simulink model "vslipsl_sim"  (R2022b)
settings: Solver=ode45  StartTime=0.0  StopTime=Tf  FixedStep=1e-3  RelTol=1e-11  AbsTol=1e-11
values from neighbouring files (symbols this model uses):
  flag_dist = 0    [main.m]    (also in main_slip_w_sw_leg.m)
  gains = [gain.K_p; gain.K_d; gain.K_p_sw; gain.K_d_sw; gain.K_p_ds; gain.K_d_ds; gain.K_v_ds]    [main.m]    (also in main_slip_w_sw_leg.m)
  init_cond = [x_M_init; y_M_init; theta_init; r_init; x_CoM_init; y_CoM_init; dx_M_init; dy_M_init; dtheta_init; dr_init; dx_CoM_init; dy_CoM_init]    [main.m]    (also in main_slip_w_sw_leg.m)
  init_f_record = 0    [main.m]    (also in main_slip_w_sw_leg.m)
  init_flag = [1; dc.col_param.foot; -dc.col_param.footPlus; x_M_init; x_CoM_ss_init; flag_ref_ob]    [main.m]    (also in main_slip_w_sw_leg.m = [1; dc.col_param.foot; -dc.col_param.footPlus; x_M_init; x_C)
  param = [L0_ss; k0_ss; m_M; m_swLeg; m_swFoot; I_swLeg; I_swFoot; L_thigh; k_swFoot; k_swLeg; theta_s0; r_s0; g; L0_ds; k0_ds]    [main.m]    (also in main_slip_w_sw_leg.m)
  ref_star_ds = [ref_star.ds.x_CoM_star,      ref_star.ds.y_CoM_star, ref_star.ds.dx_CoM_star,      ref_star.ds.del_y_CoM_star, ref_star.ds.del_dx_CoM_star,      ref_star.ds.del2_y_CoM_star]    [main.m]    (also in main_slip_w_sw_leg.m)
  ref_star_ss = [ref_star.ss.x_M_star,      ref_star.ss.y_M_star, ref_star.ss.x_swFoot_star, ref_star.ss.y_swFoot_star,      ref_star.ss.del_y_M_star, ref_star.ss.del_x_swFoot_star, ref_star.ss.del_y_swFoot_star,      ref_star.ss.del2_y_M_star, ref_star.ss.del2_x_swFoot_star, ref_star.ss.del2_y_swFoot_star,      ref_star.ss.x_CoM_star]    [main.m]    (also in main_slip_w_sw_leg.m)
  sample_time = 0.001    [main.m]    (also in main_slip_w_sw_leg.m)
libraries: simulink x1
settings Model: SimulationMode=accelerator  Creator=Pelit  LastModifiedBy=mmpel
settings SolverCC: InitialStep=1e-5  AlgebraicLoopSolver=TrustRegion
settings DataIOCC: ReturnWorkspaceOutputs=off
settings DebuggingCC: UnconnectedInputMsg=warning  UnconnectedOutputMsg=warning  UnconnectedLineMsg=warning  SFMachineParentedDataDiag=warning  ArithmeticOperatorsInVariantConditions=warning
settings ModelReferenceCC: EnableRefExpFcnMdlSchedulingChecks=on
settings SFSimCC: SimUseLocalCustomCode=off  CustomCodeUndefinedFunction=UseInterfaceOnly
settings RTWCC: RTWUseLocalCustomCode=off  DLArmComputeVersion=19.05

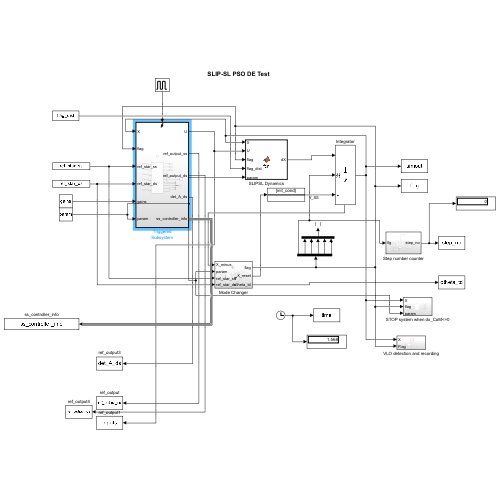
[thumbnail: Simulink's stored preview of the top-level diagram]
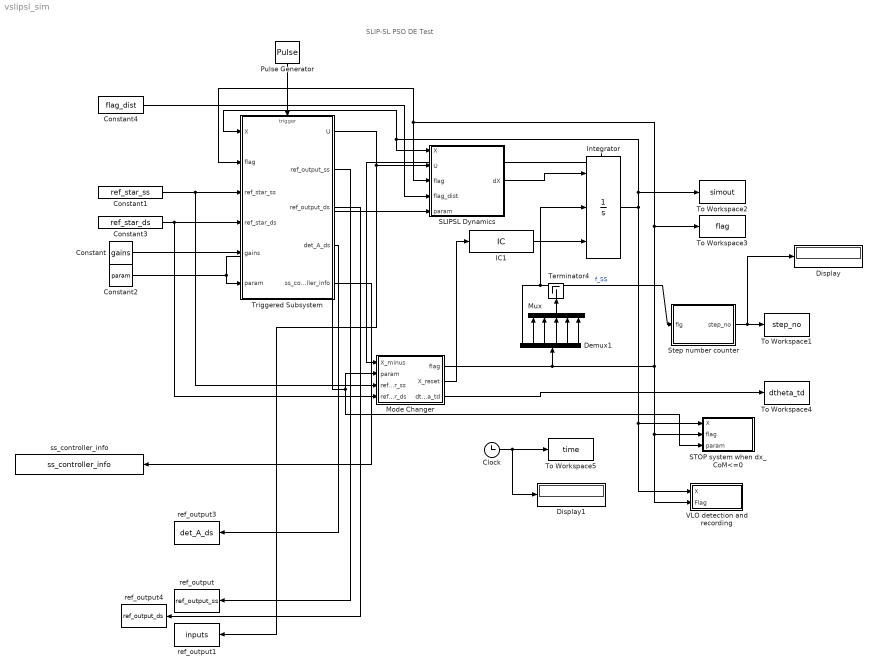
== system vslipsl_sim ==
  note: SLIP-SL PSO DE Test
  Clock : Clock
  Constant : Constant  Value=gains
  Constant1 : Constant  Value=ref_star_ss
  Constant2 : Constant  Value=param
  Constant3 : Constant  Value=ref_star_ds
  Constant4 : Constant  Value=flag_dist
  Demux1 : Demux  Outputs=6
  Display : Display
  Display1 : Display
  IC1 : InitialCondition  Value=init_cond
  Integrator : Integrator  ExternalReset=either  InitialConditionSource=external  ShowStatePort=on
  Mode Changer : Subsystem
  Mux : Mux  Inputs=5
  Pulse Generator : DiscretePulseGenerator  PulseType=Time based  Period=1e-3  PulseWidth=5
  SLIPSL Dynamics : MATLAB Function  TreatAsAtomicUnit=on
  STOP system when dx_CoM<=0 : Subsystem
  Step number counter : Subsystem
  Terminator4 : Terminator
  To Workspace1 : ToWorkspace  VariableName=step_no  SampleTime=sample_time
  To Workspace2 : ToWorkspace  VariableName=simout  SampleTime=sample_time
  To Workspace3 : ToWorkspace  VariableName=flag  SampleTime=sample_time
  To Workspace4 : ToWorkspace  VariableName=dtheta_td  SampleTime=sample_time
  To Workspace5 : ToWorkspace  VariableName=time  SampleTime=sample_time
  Triggered Subsystem : Subsystem  TreatAsAtomicUnit=on
  VLO detection and recording : Subsystem
  ref_output : ToWorkspace  VariableName=ref_output_ss  SampleTime=sample_time
  ref_output1 : ToWorkspace  VariableName=inputs  SampleTime=sample_time
  ref_output3 : ToWorkspace  VariableName=det_A_ds  SampleTime=sample_time
  ref_output4 : ToWorkspace  VariableName=ref_output_ds  SampleTime=sample_time
  ss_controller_info : ToWorkspace  VariableName=ss_controller_info  SaveFormat=Timeseries  SampleTime=sample_time
  wires:
  SLIPSL Dynamics/1(dX) -> Integrator/1
  Mode Changer/1(flag) -> Demux1/1, Triggered Subsystem/2(flag), SLIPSL Dynamics/3(flag), To Workspace3/1, VLO detection and recording/2(Flag), STOP system when dx_CoM<=0/2(flag)
  Constant2/1 -> SLIPSL Dynamics/5(param), STOP system when dx_CoM<=0/3(param), Mode Changer/2("param "), Triggered Subsystem/6(param)
  Mode Changer/2(X_reset) -> IC1/1
  Integrator/1 -> VLO detection and recording/1(X), STOP system when dx_CoM<=0/1(X), To Workspace2/1, Triggered Subsystem/1(X), SLIPSL Dynamics/1(X)
  IC1/1 -> Integrator/3
  Demux1/1 -> Step number counter/1(flg), Integrator/2  "f_SS"
  Integrator/State -> Mode Changer/1(X_minus)
  Step number counter/1(step_no) -> Display/1, To Workspace1/1
  Mode Changer/3(dtheta_td) -> To Workspace4/1
  Clock/1 -> Display1/1, To Workspace5/1
  Constant1/1 -> Mode Changer/3(ref_star_ss), Triggered Subsystem/3(ref_star_ss)
  Triggered Subsystem/1(U) -> ref_output1/1, SLIPSL Dynamics/2(U)
  Triggered Subsystem/2(ref_output_ss) -> ref_output/1
  Constant3/1 -> Mode Changer/4(ref_star_ds), Triggered Subsystem/4(ref_star_ds)
  Triggered Subsystem/3(ref_output_ds) -> ref_output4/1
  Constant/1 -> Triggered Subsystem/5(gains)
  Constant4/1 -> SLIPSL Dynamics/4(flag_dist)
  Pulse Generator/1 -> Triggered Subsystem/Trigger
  Triggered Subsystem/4(det_A_ds) -> ref_output3/1
  Demux1/2 -> Mux/1
  Demux1/3 -> Mux/2
  Demux1/4 -> Mux/3
  Demux1/5 -> Mux/4
  Demux1/6 -> Mux/5
  Mux/1 -> Terminator4/1
  Triggered Subsystem/5(ss_controller_info) -> ss_controller_info/1

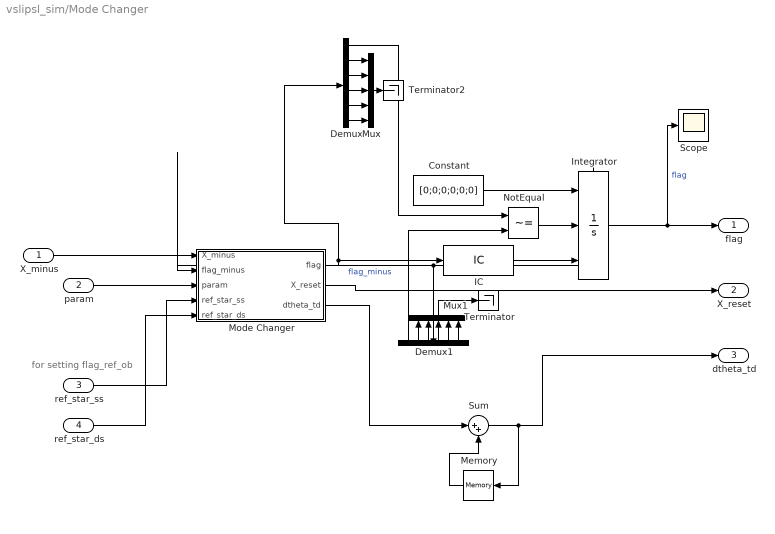
== system vslipsl_sim/Mode Changer ==
  note: for setting flag_ref_ob
  X_minus : Inport
  "param " : Inport  Port=2
  ref_star_ss : Inport  Port=3
  ref_star_ds : Inport  Port=4
  Constant : Constant  Value=[0;0;0;0;0;0]
  Demux : Demux  Outputs=6
  Demux1 : Demux  Outputs=6
  IC : InitialCondition  Value=init_flag
  Integrator : Integrator  ExternalReset=rising  InitialConditionSource=external  ShowStatePort=on
  Memory : Memory
  Mode Changer : MATLAB Function  TreatAsAtomicUnit=on
  Mux : Mux  Inputs=5
  Mux1 : Mux  Inputs=5
  NotEqual : RelationalOperator  Operator=~=  OutDataTypeStr=boolean  RndMeth=Simplest  InputSameDT=off
  Scope : Scope
  Sum : Sum  Inputs=|++
  Terminator : Terminator
  Terminator2 : Terminator
  flag : Outport  VectorParamsAs1DForOutWhenUnconnected=off
  X_reset : Outport  Port=2  VectorParamsAs1DForOutWhenUnconnected=off
  dtheta_td : Outport  Port=3  VectorParamsAs1DForOutWhenUnconnected=off
  wires:
  X_minus/1 -> Mode Changer/1(X_minus)
  IC/1 -> Integrator/3
  Integrator/State -> Mode Changer/2(flag_minus), Demux1/1  "flag_minus"
  "param "/1 -> Mode Changer/3(param)
  Mode Changer/1(flag) -> IC/1, Demux/1
  Constant/1 -> Integrator/1
  NotEqual/1 -> Integrator/2
  Integrator/1 -> Scope/1, flag/1  "flag"
  Mode Changer/2(X_reset) -> X_reset/1
  Mode Changer/3(dtheta_td) -> Sum/1
  Memory/1 -> Sum/2
  Sum/1 -> Memory/1, dtheta_td/1
  Demux1/1 -> NotEqual/2
  ref_star_ss/1 -> Mode Changer/4(ref_star_ss)
  ref_star_ds/1 -> Mode Changer/5(ref_star_ds)
  Demux/6 -> Mux/5
  Demux/5 -> Mux/4
  Demux/4 -> Mux/3
  Demux/3 -> Mux/2
  Demux/2 -> Mux/1
  Mux/1 -> Terminator2/1
  Demux/1 -> NotEqual/1
  Demux1/2 -> Mux1/1
  Demux1/3 -> Mux1/2
  Demux1/4 -> Mux1/3
  Demux1/5 -> Mux1/4
  Demux1/6 -> Mux1/5
  Mux1/1 -> Terminator/1

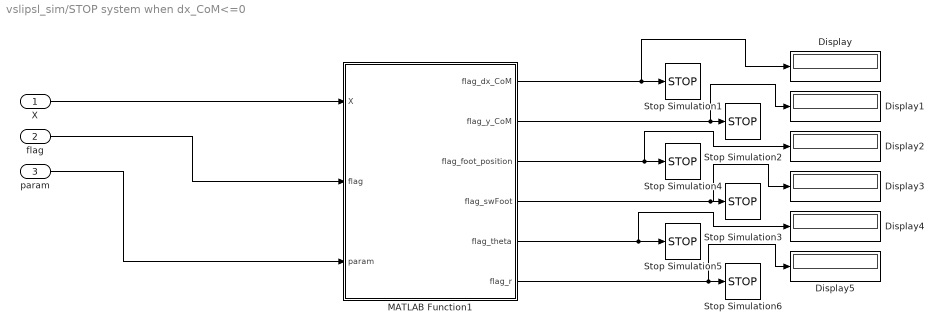
== system vslipsl_sim/STOP system when dx_CoM<=0 ==
  X : Inport
  flag : Inport  Port=2
  param : Inport  Port=3
  Display{,1..5} (6 alike) : Display
  MATLAB Function1 : MATLAB Function  TreatAsAtomicUnit=on
  Stop Simulation{1..6} (6 alike) : Stop
  wires:
  X/1 -> MATLAB Function1/1(X)
  MATLAB Function1/4(flag_swFoot) -> Display3/1, Stop Simulation3/1
  flag/1 -> MATLAB Function1/2(flag)
  param/1 -> MATLAB Function1/3(param)
  MATLAB Function1/1(flag_dx_CoM) -> Display/1, Stop Simulation1/1
  MATLAB Function1/2(flag_y_CoM) -> Display1/1, Stop Simulation2/1
  MATLAB Function1/3(flag_foot_position) -> Display2/1, Stop Simulation4/1
  MATLAB Function1/5(flag_theta) -> Display4/1, Stop Simulation5/1
  MATLAB Function1/6(flag_r) -> Display5/1, Stop Simulation6/1

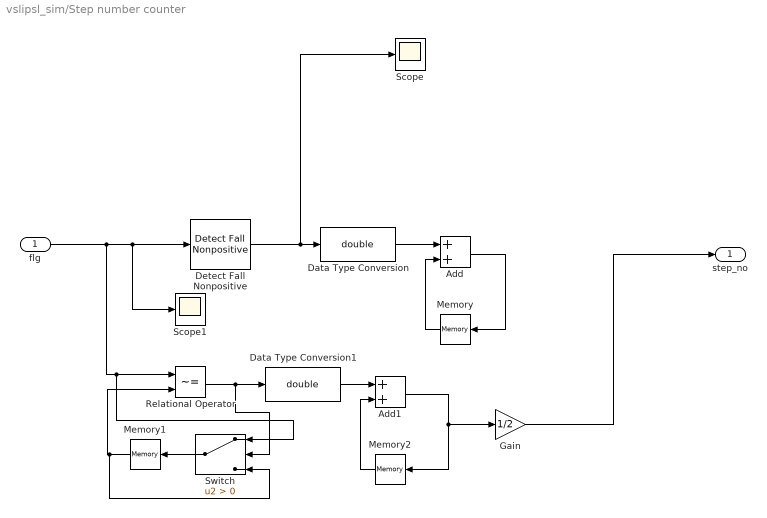
== system vslipsl_sim/Step number counter ==
  flg : Inport  SampleTime=sample_time
  Add : Sum
  Add1 : Sum
  Data Type Conversion : DataTypeConversion  OutDataTypeStr=double  SaturateOnIntegerOverflow=off  RndMeth=Floor
  Data Type Conversion1 : DataTypeConversion  OutDataTypeStr=double  SaturateOnIntegerOverflow=off  RndMeth=Floor
  Detect Fall Nonpositive : simulink/Logic and Bit Operations/Detect Fall Nonpositive  vinit=1  InputProcessing=Columns as channels (frame based)  OutDataTypeStr=boolean
  Gain : Gain  Gain=1/2
  Memory : Memory  InheritSampleTime=on
  Memory1 : Memory  InitialCondition=1  InheritSampleTime=on
  Memory2 : Memory  InheritSampleTime=on
  Relational Operator : RelationalOperator  Operator=~=  OutDataTypeStr=boolean  RndMeth=Simplest  InputSameDT=off
  Scope : Scope
  Scope1 : Scope
  Switch : Switch  Criteria=u2 > Threshold  SaturateOnIntegerOverflow=off  InputSameDT=off
  step_no : Outport  VectorParamsAs1DForOutWhenUnconnected=off
  wires:
  Add/1 -> Memory/1
  Memory/1 -> Add/2
  Detect Fall Nonpositive/1 -> Scope/1, Data Type Conversion/1
  Data Type Conversion/1 -> Add/1
  Memory1/1 -> Switch/3, Relational Operator/2
  Memory2/1 -> Add1/2
  Add1/1 -> Gain/1, Memory2/1
  Relational Operator/1 -> Switch/2, Data Type Conversion1/1
  Data Type Conversion1/1 -> Add1/1
  Switch/1 -> Memory1/1
  flg/1 -> Switch/1, Relational Operator/1, Detect Fall Nonpositive/1, Scope1/1
  Gain/1 -> step_no/1

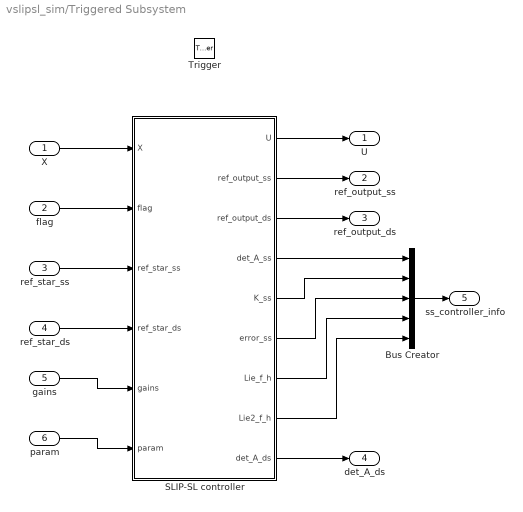
== system vslipsl_sim/Triggered Subsystem ==
  X : Inport
  flag : Inport  Port=2
  ref_star_ss : Inport  Port=3
  ref_star_ds : Inport  Port=4
  gains : Inport  Port=5
  param : Inport  Port=6
  Trigger : TriggerPort  VariantControl=Variant
  Bus Creator : BusCreator  Inputs=5
  SLIP-SL controller : MATLAB Function  TreatAsAtomicUnit=on
  U : Outport
  ref_output_ss : Outport  Port=2
  ref_output_ds : Outport  Port=3
  det_A_ds : Outport  Port=4
  ss_controller_info : Outport  Port=5
  wires:
  X/1 -> SLIP-SL controller/1(X)
  flag/1 -> SLIP-SL controller/2(flag)
  ref_star_ss/1 -> SLIP-SL controller/3(ref_star_ss)
  ref_star_ds/1 -> SLIP-SL controller/4(ref_star_ds)
  gains/1 -> SLIP-SL controller/5(gains)
  param/1 -> SLIP-SL controller/6(param)
  SLIP-SL controller/1(U) -> U/1
  SLIP-SL controller/2(ref_output_ss) -> ref_output_ss/1
  SLIP-SL controller/3(ref_output_ds) -> ref_output_ds/1
  SLIP-SL controller/4(det_A_ss) -> Bus Creator/1
  SLIP-SL controller/9(det_A_ds) -> det_A_ds/1
  Bus Creator/1 -> ss_controller_info/1
  SLIP-SL controller/5(K_ss) -> Bus Creator/2
  SLIP-SL controller/6(error_ss) -> Bus Creator/3
  SLIP-SL controller/7(Lie_f_h) -> Bus Creator/4
  SLIP-SL controller/8(Lie2_f_h) -> Bus Creator/5

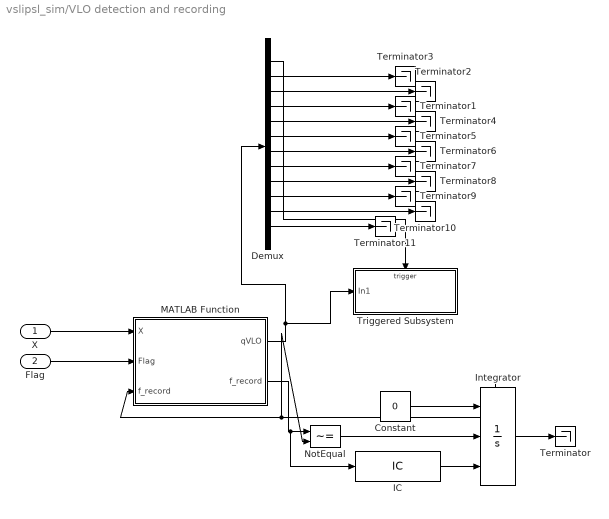
== system vslipsl_sim/VLO detection and recording ==
  X : Inport
  Flag : Inport  Port=2
  Constant : Constant  Value=0
  Demux : Demux  Outputs=12
  IC : InitialCondition  Value=init_f_record
  Integrator : Integrator  ExternalReset=rising  InitialConditionSource=external  ShowStatePort=on
  MATLAB Function : MATLAB Function  TreatAsAtomicUnit=on
  NotEqual : RelationalOperator  Operator=~=  OutDataTypeStr=boolean  RndMeth=Simplest  InputSameDT=off
  Terminator{,1..11} (12 alike) : Terminator
  Triggered Subsystem : Subsystem  TreatAsAtomicUnit=on
  wires:
  X/1 -> MATLAB Function/1(X)
  Flag/1 -> MATLAB Function/2(Flag)
  MATLAB Function/2(f_record) -> IC/1, NotEqual/1
  IC/1 -> Integrator/3
  NotEqual/1 -> Integrator/2
  Integrator/State -> MATLAB Function/3("f_record "), NotEqual/2
  Constant/1 -> Integrator/1
  Integrator/1 -> Terminator/1
  MATLAB Function/1(qVLO) -> Triggered Subsystem/1(In1), Demux/1
  Demux/1 -> Triggered Subsystem/Trigger
  Demux/2 -> Terminator3/1
  Demux/3 -> Terminator2/1
  Demux/4 -> Terminator1/1
  Demux/5 -> Terminator4/1
  Demux/6 -> Terminator5/1
  Demux/7 -> Terminator6/1
  Demux/8 -> Terminator7/1
  Demux/9 -> Terminator8/1
  Demux/10 -> Terminator9/1
  Demux/11 -> Terminator10/1
  Demux/12 -> Terminator11/1

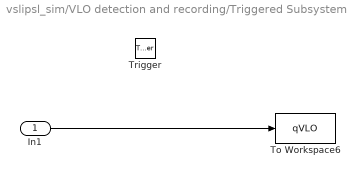
== system vslipsl_sim/VLO detection and recording/Triggered Subsystem ==
  In1 : Inport
  Trigger : TriggerPort  VariantControl=Variant
  To Workspace6 : ToWorkspace  VariableName=qVLO  SampleTime=-1
  wires:
  In1/1 -> To Workspace6/1

== matlab function vslipsl_sim/VLO detection and recording/MATLAB Function ==
  data: X input; qVLO output; Flag input; f_record output; f_record input
function [qVLO, f_record] = fcn(X, Flag, f_record)
% function for deciding when VLO occurs and records it

% ----------- states ----------------------
x_CoM = X(1); % x position of CoM
z_CoM = X(2); % z position of CoM
theta = X(3); % angle of the swing leg when in SS
r_swFoot = X(4); % distance of the foot from the knee on SS

dx_CoM = X(5); % x velocity of CoM
dz_CoM = X(6); % z velocity of CoM
dtheta = X(7);
dr_swFoot = X(8);

% ----------- flags ----------------------
f_stance = Flag(1); % indicates which stance phase it is
foot = Flag(2); % location of the stance foot
foot_prev = Flag(3); % previous location of the stance foot

% recording
if x_CoM >= foot && f_record == 0
    % this can only happen in single stance phase i.e. f_stance == 1
    qVLO = X;
    f_record = 1;
else
    qVLO = zeros(size(X));
end

% resetting the record flag
if f_record == 1 && x_CoM < foot
    f_record = 0; % when a VLO value is recorded, f_record becomes 1, then 
    % when the system goes back to double stance phase, reset the record
    % flag
end

== matlab function vslipsl_sim/Mode Changer/Mode Changer ==
  data: X_minus input; flag output; flag_minus input; param input; X_reset output; dtheta_td output; ref_star_ss input; ref_star_ds input
function [flag, X_reset, dtheta_td]  = fcn(X_minus, flag_minus, param, ref_star_ss, ref_star_ds)

% parameters
L0_ss = param(1); % [m]
k0_ss = param(2); % nominal leg stiffness [N/m]
m_M = param(3); % hip mass [kg]
m_swLeg = param(4); % [kg]
m_swFoot = param(5); % [kg]
I_swLeg = param(6); %
I_swFoot = param(7); %
L_thigh = param(8); % [m]
k_swFoot = param(9); %
k_swLeg = param(10); %
theta0 = param(11); %[rad]
r0 = param(12); % [m]
gravi = param(13); % gravitational acc

L0_ds = param(14); % [m] free length of the springs in the DS
k0_ds = param(15); % [N/m] stiffness of the springs in the DS

% flags
f_SS = flag_minus(1); % indicates which stance phase it is
foot = flag_minus(2); % location of the stance foot
foot_prev = flag_minus(3); % previous location of the stance foot
x_CoM_TD = flag_minus(4);
x_CoM_LO = flag_minus(5);
flag_ref_ob = flag_minus(6); % if the walking phase starts with reference variable out of bounds, set to true

% states
x_M = X_minus(1); % x position of CoM
y_M = X_minus(2); % z position of CoM
theta = X_minus(3); % angle of the swing leg when in SS
r = X_minus(4); % distance of the foot from the knee on SS
x_CoM = X_minus(5);
y_CoM = X_minus(6);

dx_M = X_minus(7); % x velocity of CoM
dy_M = X_minus(8); % z velocity of CoM
dtheta = X_minus(9);
dr = X_minus(10);
dx_CoM = X_minus(11);
dy_CoM = X_minus(12);

% calculating spring forces

L1 = sqrt((x_CoM - foot)^2 + y_CoM^2); % length of the new stance leg
L2 = sqrt((x_CoM - foot_prev)^2 + y_CoM^2); % length of the old stance leg

% Fs1 = k0_ds * ((L0_ds/L1) - 1) * [x_CoM - foot; y_CoM]; % Spring force of the new stance leg
Fs2 = k0_ds * ((L0_ds/L2 )- 1) * [x_CoM - foot_prev; y_CoM]; % Spring force of the old stance leg

sw_foot_x = x_M + (L_thigh + r)*cos(theta);
sw_foot_y = y_M + (L_thigh + r)*sin(theta); % y position of the swing foot

dy_swFoot = dy_M + dr*sin(theta) + (L_thigh + r)*cos(theta)*dtheta;

X_reset = [0;0.9800;0.7854;0;0.1000;0.9800;0;0; 0; 0; 0; 0]; % dummy X_reset so that simulink doesn't give error

dtheta_td = 0;

%% reference trajectory phase variables
x_CoM_star_ss = ref_star_ss(:,11);
x_CoM_star_ds = ref_star_ds(:,1);

%%

% if f_SS == 1 && sw_foot_y <= 0 && dy_swFoot < 0
if f_SS == 1 && sw_foot_y <= 0 && sw_foot_x > x_M
    % change from single stance phase to double stance phase
    f_SS = -1;
    foot_prev = foot; % saving the old foot location
    foot = sw_foot_x; % calculating the new foots location
    
    dtheta_td = dtheta; % leg speed at the moment of touchdown
    
    % CoM position and velocities when SLIP-SL becomes SLIP in the double
    % stance phase
    
    x_CoM_plus = (m_swLeg*(x_M + (L_thigh*cos(theta))/2) + m_M*x_M + m_swFoot*(x_M + cos(theta)*(L_thigh + r)))/(m_M + m_swLeg + m_swFoot);
    y_CoM_plus = (m_swFoot*(y_M + sin(theta)*(L_thigh + r)) + m_swLeg*(y_M + (L_thigh*sin(theta))/2) + m_M*y_M)/(m_M + m_swLeg + m_swFoot);
    
    dx_CoM_plus = dx_M + (dr*m_swFoot*cos(theta))/(m_M + m_swLeg + m_swFoot) - (dtheta*sin(theta)*((L_thigh*m_swLeg)/2 + L_thigh*m_swFoot + m_swFoot*r))/(m_M + m_swLeg + m_swFoot);
    dy_CoM_plus = dy_M + (dr*m_swFoot*sin(theta))/(m_M + m_swLeg + m_swFoot) + (dtheta*cos(theta)*((L_thigh*m_swLeg)/2 + L_thigh*m_swFoot + m_swFoot*r))/(m_M + m_swLeg + m_swFoot);
    
    X_reset = [
        0; 0; 0; 0; x_CoM_plus; y_CoM_plus;
        0; 0; 0; 0; dx_CoM_plus; dy_CoM_plus];

    x_CoM_TD = x_CoM_plus;

    % check if the phase variable is out of bounds and raise the flag is so
    if x_CoM_plus - foot < x_CoM_star_ds(1)
        flag_ref_ob = 1;
    else
        flag_ref_ob = 0;
    end
    
elseif f_SS == -1 && Fs2(2) <= 0
    % change from double stance phase to single stance phase
    f_SS = 1;
    
    
    F_X = @(X) [
        x_CoM - (m_swFoot*(X(1) + cos(X(3))*(L_thigh + X(4))) + m_swLeg*(X(1) + (L_thigh*cos(X(3)))/2) + m_M*X(1))/(m_M + m_swLeg + m_swFoot);
        y_CoM - (m_swFoot*(X(2) + sin(X(3))*(L_thigh + X(4))) + m_swLeg*(X(2) + (L_thigh*sin(X(3)))/2) + m_M*X(2))/(m_M + m_swLeg + m_swFoot);
        X(1) - foot_prev + cos(X(3))*(L_thigh + X(4));
        X(2) + sin(X(3))*(L_thigh + X(4))];
    
    %options = optimoptions('Algorithm', 'Levenberg-Marquardt');
    X_plus = fsolve(F_X,[x_CoM,1.0479,4.5052,0.3708],optimoptions('fsolve','Algorithm', 'Levenberg-Marquardt'));
    
    theta_plus = X_plus(3);
    r_plus = X_plus(4);
    
    F_dX = @(dX) [
        dx_CoM - (dX(1)*m_M + m_swLeg*(dX(1) - (L_thigh*dX(3)*sin(theta_plus))/2) + m_swFoot*(dX(1) + dX(4)*cos(theta_plus) - dX(3)*sin(theta_plus)*(L_thigh + r_plus)))/(m_M + m_swLeg + m_swFoot);
        dy_CoM - (dX(2)*m_M + m_swLeg*(dX(2) + (L_thigh*dX(3)*cos(theta_plus))/2) + m_swFoot*(dX(2) + dX(4)*sin(theta_plus) + dX(3)*cos(theta_plus)*(L_thigh + r_plus)))/(m_M + m_swLeg + m_swFoot);
        dX(1) + dX(4)*cos(theta_plus) - dX(3)*sin(theta_plus)*(L_thigh + r_plus);
        dX(2) + dX(4)*sin(theta_plus) + dX(3)*cos(theta_plus)*(L_thigh + r_plus)];
    
    dX_plus = fsolve(F_dX, [0.7156,0.1696,-0.6214,0.3132], optimoptions('fsolve','Algorithm', 'Levenberg-Marquardt'));
    
    
    X_reset = [
        X_plus(1); X_plus(2); X_plus(3); X_plus(4); x_CoM; y_CoM;
        dX_plus(1); dX_plus(2); dX_plus(3); dX_plus(4); dx_CoM; dy_CoM];
    
    x_M_LO = X_plus(1) - foot; % recording the x_M @LO relative to foot
    theta_LO = X_plus(3);
    r_LO = X_plus(4);
    
    x_swLeg_LO = x_M_LO + (L_thigh/2)*cos(theta_LO);
    x_swFoot_LO = x_M_LO + (L_thigh + r_LO)*cos(theta_LO);
    
    x_CoM_LO = (m_M*x_M_LO + m_swLeg*x_swLeg_LO + m_swFoot*x_swFoot_LO)/(m_M + m_swLeg + m_swFoot); % recording the x_CoM @LO relative to foot

    % check if the phase variable is out of bounds and raise the flag is so
    if x_CoM_LO < x_CoM_star_ss(1)
        flag_ref_ob = 1;
    else
        flag_ref_ob = 0;
    end
    
end

flag = [f_SS; foot; foot_prev; x_CoM_TD; x_CoM_LO; flag_ref_ob];

== matlab function vslipsl_sim/SLIPSL Dynamics ==
  data: X input; U input; dX output; flag input; flag_dist input; param input
function dX  = fcn(X, U, flag, flag_dist, param)

% ----------- parameters ----------------------
L0_ss = param(1); % [m]
k0_ss = param(2); % nominal leg stiffness [N/m]
m_M = param(3); % hip mass [kg]
m_swLeg = param(4); % [kg]
m_swFoot = param(5); % [kg]
I_swLeg = param(6); %
I_swFoot = param(7); %
L_thigh = param(8); % [m]
k_swFoot = param(9); %
k_swLeg = param(10); %
theta0 = param(11); %[rad]
r0 = param(12); % [m]
gravi = param(13); % gravitational acc

L0_ds = param(14); % [m] free length of the springs in the DS
k0_ds = param(15); % [N/m] stiffness of the springs in the DS

% ----------- flags ----------------------
f_stance = flag(1); % indicates which stance phase it is
foot = flag(2); % location of the stance foot
foot_prev = flag(3); % previous location of the stance foot

% ----------- states ----------------------
x_M = X(1); % x position of main mass in SS
y_M = X(2); % z position of main mass in SS
theta = X(3); % angle of the swing leg when in SS
r = X(4); % distance of the foot from the knee on SS
x_CoM = X(5); % x position of the CoM
y_CoM = X(6);

dx_M = X(7); % x velocity of main mass in SS
dy_M = X(8); % z velocity of main mass in SS
dtheta = X(9);
dr = X(10);
dx_CoM = X(11);
dy_CoM = X(12);

q = [x_M; y_M; theta; r; x_CoM; y_CoM];
dq = [dx_M; dy_M; dtheta; dr; dx_CoM; dy_CoM];

% --------- controller ---------------------

u1 = U(1);
u2 = U(2);
u3 = U(3);
u4 = U(4);
u5 = U(5);

% -------- disturbance ---------------------------
if x_CoM >= 1.0 && x_CoM <= 1.01 && flag_dist == 1
    F_dist = [-45;60; 0; 0];
else
    F_dist = [0; 0; 0; 0];
end

% ----------- calculation of acceleration ----------------------
if f_stance == 1
    % single stance phase
    
%     % controller actions
%     
%     k0_ss = k0_ss + u1;
%     k_swLeg = k_swLeg + u2;
%     k_swFoot = k_swFoot + u3;
% 
%     % generalized accelerations obtained from derivation_of_DE.m
%     ddq1 = ((foot*k0_ss - k0_ss*x_M - (L0_ss*foot*k0_ss)/(y_M^2 + (foot - x_M)^2)^(1/2) + (L0_ss*k0_ss*x_M)/(y_M^2 + (foot - x_M)^2)^(1/2) + 2*dr*dtheta*m_swFoot*sin(theta) + (L_thigh*dtheta^2*m_swLeg*cos(theta))/2 + L_thigh*dtheta^2*m_swFoot*cos(theta) + dtheta^2*m_swFoot*r*cos(theta))*(4*I_swLeg*m_M + 4*I_swFoot*m_M + 4*I_swLeg*m_swLeg + 4*I_swLeg*m_swFoot + 4*I_swFoot*m_swLeg + 4*I_swFoot*m_swFoot + 4*m_M*m_swFoot*r^2 + 4*m_swLeg*m_swFoot*r^2 + L_thigh^2*m_swLeg^2*sin(theta)^2 - 4*I_swLeg*m_swFoot*sin(theta)^2 - 4*I_swFoot*m_swFoot*sin(theta)^2 + L_thigh^2*m_M*m_swLeg + 4*L_thigh^2*m_M*m_swFoot + L_thigh^2*m_swLeg*m_swFoot + 3*L_thigh^2*m_swLeg*m_swFoot*sin(theta)^2 + 8*L_thigh*m_M*m_swFoot*r + 4*L_thigh*m_swLeg*m_swFoot*r + 4*L_thigh*m_swLeg*m_swFoot*r*sin(theta)^2))/((m_M + m_swLeg)*(4*I_swLeg*m_M + 4*I_swFoot*m_M + 4*I_swLeg*m_swLeg + 4*I_swLeg*m_swFoot + 4*I_swFoot*m_swLeg + 4*I_swFoot*m_swFoot + 4*m_M*m_swFoot*r^2 + 4*m_swLeg*m_swFoot*r^2 + L_thigh^2*m_M*m_swLeg + 4*L_thigh^2*m_M*m_swFoot + L_thigh^2*m_swLeg*m_swFoot + 8*L_thigh*m_M*m_swFoot*r + 4*L_thigh*m_swLeg*m_swFoot*r)) - (((L_thigh*m_swLeg)/2 + L_thigh*m_swFoot + m_swFoot*r)*(4*k_swLeg*theta*sin(theta) - 4*k_swLeg*theta0*sin(theta) + L_thigh*gravi*m_swLeg*sin(2*theta) + 2*L_thigh*gravi*m_swFoot*sin(2*theta) + 2*gravi*m_swFoot*r*sin(2*theta) + 8*L_thigh*dr*dtheta*m_swFoot*sin(theta) + 8*dr*dtheta*m_swFoot*r*sin(theta)))/(4*I_swLeg*m_M + 4*I_swFoot*m_M + 4*I_swLeg*m_swLeg + 4*I_swLeg*m_swFoot + 4*I_swFoot*m_swLeg + 4*I_swFoot*m_swFoot + 4*m_M*m_swFoot*r^2 + 4*m_swLeg*m_swFoot*r^2 + L_thigh^2*m_M*m_swLeg + 4*L_thigh^2*m_M*m_swFoot + L_thigh^2*m_swLeg*m_swFoot + 8*L_thigh*m_M*m_swFoot*r + 4*L_thigh*m_swLeg*m_swFoot*r) - (k_swFoot*r0*cos(theta) - k_swFoot*r*cos(theta) - (gravi*m_swFoot*sin(2*theta))/2 + L_thigh*dtheta^2*m_swFoot*cos(theta) + dtheta^2*m_swFoot*r*cos(theta))/(m_M + m_swLeg) - (2*cos(theta)*sin(theta)*((L_thigh^2*m_swLeg^2)/2 + (3*m_swFoot*L_thigh^2*m_swLeg)/2 + 2*m_swFoot*r*L_thigh*m_swLeg - 2*I_swLeg*m_swFoot - 2*I_swFoot*m_swFoot)*((L0_ss*k0_ss*y_M)/(y_M^2 + (foot - x_M)^2)^(1/2) - gravi*(m_M + m_swLeg + m_swFoot) - k0_ss*y_M - 2*dr*dtheta*m_swFoot*cos(theta) + (L_thigh*dtheta^2*m_swLeg*sin(theta))/2 + L_thigh*dtheta^2*m_swFoot*sin(theta) + dtheta^2*m_swFoot*r*sin(theta)))/((m_M + m_swLeg)*(4*I_swLeg*m_M + 4*I_swFoot*m_M + 4*I_swLeg*m_swLeg + 4*I_swLeg*m_swFoot + 4*I_swFoot*m_swLeg + 4*I_swFoot*m_swFoot + 4*m_M*m_swFoot*r^2 + 4*m_swLeg*m_swFoot*r^2 + L_thigh^2*m_M*m_swLeg + 4*L_thigh^2*m_M*m_swFoot + L_thigh^2*m_swLeg*m_swFoot + 8*L_thigh*m_M*m_swFoot*r + 4*L_thigh*m_swLeg*m_swFoot*r));
%     ddq2 = (((L0_ss*k0_ss*y_M)/(y_M^2 + (foot - x_M)^2)^(1/2) - gravi*(m_M + m_swLeg + m_swFoot) - k0_ss*y_M - 2*dr*dtheta*m_swFoot*cos(theta) + (L_thigh*dtheta^2*m_swLeg*sin(theta))/2 + L_thigh*dtheta^2*m_swFoot*sin(theta) + dtheta^2*m_swFoot*r*sin(theta))*(4*I_swLeg*m_M + 4*I_swFoot*m_M + 4*I_swLeg*m_swLeg + 4*I_swFoot*m_swLeg + L_thigh^2*m_swLeg^2 + 4*m_M*m_swFoot*r^2 + 4*m_swLeg*m_swFoot*r^2 - L_thigh^2*m_swLeg^2*sin(theta)^2 + 4*I_swLeg*m_swFoot*sin(theta)^2 + 4*I_swFoot*m_swFoot*sin(theta)^2 + L_thigh^2*m_M*m_swLeg + 4*L_thigh^2*m_M*m_swFoot + 4*L_thigh^2*m_swLeg*m_swFoot - 3*L_thigh^2*m_swLeg*m_swFoot*sin(theta)^2 + 8*L_thigh*m_M*m_swFoot*r + 8*L_thigh*m_swLeg*m_swFoot*r - 4*L_thigh*m_swLeg*m_swFoot*r*sin(theta)^2))/((m_M + m_swLeg)*(4*I_swLeg*m_M + 4*I_swFoot*m_M + 4*I_swLeg*m_swLeg + 4*I_swLeg*m_swFoot + 4*I_swFoot*m_swLeg + 4*I_swFoot*m_swFoot + 4*m_M*m_swFoot*r^2 + 4*m_swLeg*m_swFoot*r^2 + L_thigh^2*m_M*m_swLeg + 4*L_thigh^2*m_M*m_swFoot + L_thigh^2*m_swLeg*m_swFoot + 8*L_thigh*m_M*m_swFoot*r + 4*L_thigh*m_swLeg*m_swFoot*r)) - (sin(theta)*(k_swFoot*r0 - k_swFoot*r + dtheta^2*m_swFoot*r - gravi*m_swFoot*sin(theta) + L_thigh*dtheta^2*m_swFoot))/(m_M + m_swLeg) + (cos(theta)*(L_thigh*m_swLeg + 2*L_thigh*m_swFoot + 2*m_swFoot*r)*(2*k_swLeg*theta - 2*k_swLeg*theta0 + 4*dr*dtheta*m_swFoot*r + L_thigh*gravi*m_swLeg*cos(theta) + 2*L_thigh*gravi*m_swFoot*cos(theta) + 2*gravi*m_swFoot*r*cos(theta) + 4*L_thigh*dr*dtheta*m_swFoot))/(4*I_swLeg*m_M + 4*I_swFoot*m_M + 4*I_swLeg*m_swLeg + 4*I_swLeg*m_swFoot + 4*I_swFoot*m_swLeg + 4*I_swFoot*m_swFoot + 4*m_M*m_swFoot*r^2 + 4*m_swLeg*m_swFoot*r^2 + L_thigh^2*m_M*m_swLeg + 4*L_thigh^2*m_M*m_swFoot + L_thigh^2*m_swLeg*m_swFoot + 8*L_thigh*m_M*m_swFoot*r + 4*L_thigh*m_swLeg*m_swFoot*r) - (2*cos(theta)*sin(theta)*((L_thigh^2*m_swLeg^2)/2 + (3*m_swFoot*L_thigh^2*m_swLeg)/2 + 2*m_swFoot*r*L_thigh*m_swLeg - 2*I_swLeg*m_swFoot - 2*I_swFoot*m_swFoot)*(foot*k0_ss - k0_ss*x_M - (L0_ss*foot*k0_ss)/(y_M^2 + (foot - x_M)^2)^(1/2) + (L0_ss*k0_ss*x_M)/(y_M^2 + (foot - x_M)^2)^(1/2) + 2*dr*dtheta*m_swFoot*sin(theta) + (L_thigh*dtheta^2*m_swLeg*cos(theta))/2 + L_thigh*dtheta^2*m_swFoot*cos(theta) + dtheta^2*m_swFoot*r*cos(theta)))/((m_M + m_swLeg)*(4*I_swLeg*m_M + 4*I_swFoot*m_M + 4*I_swLeg*m_swLeg + 4*I_swLeg*m_swFoot + 4*I_swFoot*m_swLeg + 4*I_swFoot*m_swFoot + 4*m_M*m_swFoot*r^2 + 4*m_swLeg*m_swFoot*r^2 + L_thigh^2*m_M*m_swLeg + 4*L_thigh^2*m_M*m_swFoot + L_thigh^2*m_swLeg*m_swFoot + 8*L_thigh*m_M*m_swFoot*r + 4*L_thigh*m_swLeg*m_swFoot*r));
%     ddq3 = -(4*k_swLeg*m_M*theta*(foot^2 - 2*foot*x_M + x_M^2 + y_M^2)^(1/2) - 4*k_swLeg*m_M*theta0*(foot^2 - 2*foot*x_M + x_M^2 + y_M^2)^(1/2) + 4*k_swLeg*m_swLeg*theta*(foot^2 - 2*foot*x_M + x_M^2 + y_M^2)^(1/2) - 4*k_swLeg*m_swLeg*theta0*(foot^2 - 2*foot*x_M + x_M^2 + y_M^2)^(1/2) + 4*k_swLeg*m_swFoot*theta*(foot^2 - 2*foot*x_M + x_M^2 + y_M^2)^(1/2) - 4*k_swLeg*m_swFoot*theta0*(foot^2 - 2*foot*x_M + x_M^2 + y_M^2)^(1/2) + 2*L0_ss*L_thigh*foot*k0_ss*m_swLeg*sin(theta) + 4*L0_ss*L_thigh*foot*k0_ss*m_swFoot*sin(theta) + 2*L0_ss*L_thigh*k0_ss*m_swLeg*y_M*cos(theta) + 4*L0_ss*L_thigh*k0_ss*m_swFoot*y_M*cos(theta) - 2*L0_ss*L_thigh*k0_ss*m_swLeg*x_M*sin(theta) - 4*L0_ss*L_thigh*k0_ss*m_swFoot*x_M*sin(theta) + 4*L0_ss*foot*k0_ss*m_swFoot*r*sin(theta) - 2*L_thigh*foot*k0_ss*m_swLeg*sin(theta)*(foot^2 - 2*foot*x_M + x_M^2 + y_M^2)^(1/2) - 4*L_thigh*foot*k0_ss*m_swFoot*sin(theta)*(foot^2 - 2*foot*x_M + x_M^2 + y_M^2)^(1/2) + 4*L0_ss*k0_ss*m_swFoot*r*y_M*cos(theta) - 2*L_thigh*k0_ss*m_swLeg*y_M*cos(theta)*(foot^2 - 2*foot*x_M + x_M^2 + y_M^2)^(1/2) - 4*L_thigh*k0_ss*m_swFoot*y_M*cos(theta)*(foot^2 - 2*foot*x_M + x_M^2 + y_M^2)^(1/2) - 4*L0_ss*k0_ss*m_swFoot*r*x_M*sin(theta) + 2*L_thigh*k0_ss*m_swLeg*x_M*sin(theta)*(foot^2 - 2*foot*x_M + x_M^2 + y_M^2)^(1/2) + 4*L_thigh*k0_ss*m_swFoot*x_M*sin(theta)*(foot^2 - 2*foot*x_M + x_M^2 + y_M^2)^(1/2) - 4*foot*k0_ss*m_swFoot*r*sin(theta)*(foot^2 - 2*foot*x_M + x_M^2 + y_M^2)^(1/2) - 4*k0_ss*m_swFoot*r*y_M*cos(theta)*(foot^2 - 2*foot*x_M + x_M^2 + y_M^2)^(1/2) + 4*k0_ss*m_swFoot*r*x_M*sin(theta)*(foot^2 - 2*foot*x_M + x_M^2 + y_M^2)^(1/2) + 8*L_thigh*dr*dtheta*m_M*m_swFoot*(foot^2 - 2*foot*x_M + x_M^2 + y_M^2)^(1/2) + 4*L_thigh*dr*dtheta*m_swLeg*m_swFoot*(foot^2 - 2*foot*x_M + x_M^2 + y_M^2)^(1/2) + 8*dr*dtheta*m_M*m_swFoot*r*(foot^2 - 2*foot*x_M + x_M^2 + y_M^2)^(1/2) + 8*dr*dtheta*m_swLeg*m_swFoot*r*(foot^2 - 2*foot*x_M + x_M^2 + y_M^2)^(1/2))/((foot^2 - 2*foot*x_M + x_M^2 + y_M^2)^(1/2)*(4*I_swLeg*m_M + 4*I_swFoot*m_M + 4*I_swLeg*m_swLeg + 4*I_swLeg*m_swFoot + 4*I_swFoot*m_swLeg + 4*I_swFoot*m_swFoot + 4*m_M*m_swFoot*r^2 + 4*m_swLeg*m_swFoot*r^2 + L_thigh^2*m_M*m_swLeg + 4*L_thigh^2*m_M*m_swFoot + L_thigh^2*m_swLeg*m_swFoot + 8*L_thigh*m_M*m_swFoot*r + 4*L_thigh*m_swLeg*m_swFoot*r));
%     ddq4 = ((m_M + m_swLeg + m_swFoot)*(k_swFoot*r0 - k_swFoot*r + dtheta^2*m_swFoot*r - gravi*m_swFoot*sin(theta) + L_thigh*dtheta^2*m_swFoot))/(m_swFoot*(m_M + m_swLeg)) - (sin(theta)*((L0_ss*k0_ss*y_M)/(y_M^2 + (foot - x_M)^2)^(1/2) - gravi*(m_M + m_swLeg + m_swFoot) - k0_ss*y_M - 2*dr*dtheta*m_swFoot*cos(theta) + (L_thigh*dtheta^2*m_swLeg*sin(theta))/2 + L_thigh*dtheta^2*m_swFoot*sin(theta) + dtheta^2*m_swFoot*r*sin(theta)))/(m_M + m_swLeg) - (cos(theta)*(foot*k0_ss - k0_ss*x_M - (L0_ss*foot*k0_ss)/(y_M^2 + (foot - x_M)^2)^(1/2) + (L0_ss*k0_ss*x_M)/(y_M^2 + (foot - x_M)^2)^(1/2) + 2*dr*dtheta*m_swFoot*sin(theta) + (L_thigh*dtheta^2*m_swLeg*cos(theta))/2 + L_thigh*dtheta^2*m_swFoot*cos(theta) + dtheta^2*m_swFoot*r*cos(theta)))/(m_M + m_swLeg);
%     
%     % Time Derivative of CoM, this is directly calculated from first 4
%     % generalized coordinates
%     ddx_M = ddq1;
%     ddy_M = ddq2;
%     ddtheta = ddq3; 
%     ddr = ddq4;
%     
%     ddq5 = ddx_M + (ddr*cos(theta))/18 - (dr*dtheta*sin(theta))/9 - (ddtheta*r*sin(theta))/18 - (L_thigh*dtheta^2*cos(theta))/12 - (dtheta^2*r*cos(theta))/18 - (L_thigh*ddtheta*sin(theta))/12;
%     ddq6 = ddy_M + (ddr*sin(theta))/18 + (dr*dtheta*cos(theta))/9 + (ddtheta*r*cos(theta))/18 - (L_thigh*dtheta^2*sin(theta))/12 - (dtheta^2*r*sin(theta))/18 + (L_thigh*ddtheta*cos(theta))/12;
%     
%     dq = [dx_M; dy_M; dtheta; dr; dx_CoM; dy_CoM];
%     ddq = [ddq1; ddq2; ddq3; ddq4; ddq5; ddq6];

    M = [
                                                     m_M + m_swLeg + m_swFoot,                                                                    0,                                 -(sin(theta)*(L_thigh*m_swLeg + 2*L_thigh*m_swFoot + 2*m_swFoot*r))/2, m_swFoot*cos(theta);
                                                                            0,                                             m_M + m_swLeg + m_swFoot,                                  (cos(theta)*(L_thigh*m_swLeg + 2*L_thigh*m_swFoot + 2*m_swFoot*r))/2, m_swFoot*sin(theta);
        -(sin(theta)*(L_thigh*m_swLeg + 2*L_thigh*m_swFoot + 2*m_swFoot*r))/2, (cos(theta)*(L_thigh*m_swLeg + 2*L_thigh*m_swFoot + 2*m_swFoot*r))/2, I_swLeg + I_swFoot + (L_thigh^2*m_swLeg)/4 + L_thigh^2*m_swFoot + m_swFoot*r^2 + 2*L_thigh*m_swFoot*r,                   0;
                                                          m_swFoot*cos(theta),                                                  m_swFoot*sin(theta),                                                                                                     0,            m_swFoot];
                                                      
    C = [
        k0_ss*x_M - foot*k0_ss + (L0_ss*foot*k0_ss)/(y_M^2 + (foot - x_M)^2)^(1/2) - (L0_ss*k0_ss*x_M)/(y_M^2 + (foot - x_M)^2)^(1/2) - 2*dr*dtheta*m_swFoot*sin(theta) - (L_thigh*dtheta^2*m_swLeg*cos(theta))/2 - L_thigh*dtheta^2*m_swFoot*cos(theta) - dtheta^2*m_swFoot*r*cos(theta);
                                                                        k0_ss*y_M - (L0_ss*k0_ss*y_M)/(y_M^2 + (foot - x_M)^2)^(1/2) + 2*dr*dtheta*m_swFoot*cos(theta) - (L_thigh*dtheta^2*m_swLeg*sin(theta))/2 - L_thigh*dtheta^2*m_swFoot*sin(theta) - dtheta^2*m_swFoot*r*sin(theta);
                                                                                                                                                                                                   k_swLeg*theta - k_swLeg*theta0 + 2*dr*dtheta*m_swFoot*r + 2*L_thigh*dr*dtheta*m_swFoot;
                                                                                                                                                                                                               k_swFoot*r - k_swFoot*r0 - dtheta^2*m_swFoot*r - L_thigh*dtheta^2*m_swFoot];
                                                                                                                                                                                                           
    G = [
                                                                             0;
                                              (m_M + m_swLeg + m_swFoot)*gravi;
        gravi*cos(theta)*((L_thigh*m_swLeg)/2 + L_thigh*m_swFoot + m_swFoot*r);
                                                     m_swFoot*sin(theta)*gravi];
                                                 
    S = [
        ((foot - x_M)*(L0_ss - (y_M^2 + (foot - x_M)^2)^(1/2)))/(y_M^2 + (foot - x_M)^2)^(1/2),              0,      0;
                -(y_M*(L0_ss - (y_M^2 + (foot - x_M)^2)^(1/2)))/(y_M^2 + (foot - x_M)^2)^(1/2),              0,      0;
                                                                                             0, theta - theta0,      0;
                                                                                             0,              0, r - r0];
    U = [u1; u2; u3];
    
    % M*ddq + H = S*U
    ddq_ss = inv(M)*(-C - G -S*U + F_dist);
    
    % Time Derivative of CoM, this is directly calculated from first 4
    % generalized coordinates
    ddx_M = ddq_ss(1);
    ddy_M = ddq_ss(2);
    ddtheta = ddq_ss(3); 
    ddr = ddq_ss(4);
    ddq5 = ddx_M + (ddr*cos(theta))/18 - (dr*dtheta*sin(theta))/9 - (ddtheta*r*sin(theta))/18 - (L_thigh*dtheta^2*cos(theta))/12 - (dtheta^2*r*cos(theta))/18 - (L_thigh*ddtheta*sin(theta))/12;
    ddq6 = ddy_M + (ddr*sin(theta))/18 + (dr*dtheta*cos(theta))/9 + (ddtheta*r*cos(theta))/18 - (L_thigh*dtheta^2*sin(theta))/12 - (dtheta^2*r*sin(theta))/18 + (L_thigh*ddtheta*cos(theta))/12;
    
    
    dq = [dx_M; dy_M; dtheta; dr; dx_CoM; dy_CoM];
    ddq = [ddq_ss; ddq5; ddq6];
    
else
    % double stance phase if flag == 0
    % simple SLIP model
    L1 = sqrt((x_CoM - foot)^2 + y_CoM^2); % length of the new stance leg
    L2 = sqrt((x_CoM - foot_prev)^2 + y_CoM^2); % length of the old stance leg
    
    Fs1 = (k0_ds + u4) * ((L0_ds/L1) - 1) * [x_CoM - foot; y_CoM]; % Spring force of the new stance leg
    Fs2 = (k0_ds + u5) * ((L0_ds/L2 )- 1) * [x_CoM - foot_prev; y_CoM]; % Spring force of the old stance leg
    F = Fs1 + Fs2; % spring force matrix
    
    dq = [0; 0; 0; 0; dx_CoM; dy_CoM];
    
    ddq = [
        0;
        0;
        0;
        0;
        (F(1) + F_dist(1))/(m_M + m_swLeg + m_swFoot);
        (F(2) - (m_M + m_swLeg + m_swFoot)*gravi + F_dist(2))/(m_M + m_swLeg + m_swFoot)];
end

dX = [dq; ddq];

== matlab function vslipsl_sim/STOP system when dx_CoM<=0/MATLAB Function1 ==
  data: flag_dx_CoM output; flag_y_CoM output; flag_foot_position output; X input; flag_swFoot output; flag input; param input; flag_theta output; flag_r output
function [flag_dx_CoM, flag_y_CoM, flag_foot_position, flag_swFoot, flag_theta, flag_r] = fcn(X, flag, param)
% this function checks if the simulation is running within the constraints
% and if not, it sets related flags to 1 in order to stop the simulation

% ----------- parameters ----------------------
L0_ss = param(1); % [m]
k0_ss = param(2); % nominal leg stiffness [N/m]
m_M = param(3); % hip mass [kg]
m_swLeg = param(4); % [kg]
m_swFoot = param(5); % [kg]
I_swLeg = param(6); %
I_swFoot = param(7); %
L_thigh = param(8); % [m]
k_swFoot = param(9); %
k_swLeg = param(10); %
theta0 = param(11); %[rad]
r0 = param(12); % [m]
gravi = param(13); % gravitational acc

L0_ds = param(14); % [m] free length of the springs in the DS
k0_ds = param(15); % [N/m] stiffness of the springs in the DS

% ----------- flags ----------------------
f_stance = flag(1); % indicates which stance phase it is
foot = flag(2); % location of the stance foot
foot_prev = flag(3) - foot; % previous location of the stance foot
x_CoM_TD = flag(4); % x_CoM @TD

% ----------- states ----------------------
x_M = X(1) - foot; % x position of main mass in SS
y_M = X(2); % z position of main mass in SS
theta = X(3); % angle of the swing leg when in SS
r = X(4); % distance of the foot from the knee on SS
x_CoM = X(5) - foot; % x position of the CoM
y_CoM = X(6);

dx_M = X(7); % x velocity of main mass in SS
dy_M = X(8); % z velocity of main mass in SS
dtheta = X(9);
dr = X(10);
dx_CoM = X(11);
dy_CoM = X(12);


y_swFoot = y_M + (L_thigh + r)*sin(theta);

flag_dx_CoM = 0;
flag_y_CoM = 0;
flag_foot_position = 0;
flag_swFoot = 0;
flag_theta = 0;
flag_r = 0;

if f_stance == 1
    % check if the CoM horizontal velocity is forward
    
    % checks if foot positioning is correct
    if foot_prev >= foot
        flag_foot_position = 1;
    else
        flag_foot_position = 0;
    end
    
    % check if the swing foot is below the ground in the SS phase
    if f_stance == 1 && y_swFoot < -0.1
        flag_swFoot = 1;
    else
        flag_swFoot = 0;
    end
    
    % checks if 180<theta<360 in th SS
    if f_stance == 1 && (theta > 2*pi || theta < pi)
        flag_theta = 1;
    else
        flag_theta = 0;
    end
    
    % checks if -0.3<r<0.3 in SS
    if f_stance == 1 && (r > 0.6 || r < -0.6)
        flag_r = 1;
    else
        flag_r = 0;
    end
    
else
    % check if the CoM horizontal velocity is forward
    if dx_CoM < 0
        flag_dx_CoM = 1;
    else
        flag_dx_CoM = 0;
    end
    
    % checks if the CoM height is within proper limits
    if y_CoM > 1 || y_CoM < 0.5
        flag_y_CoM = 1;
    else
        flag_y_CoM = 0;
    end
    
    % checks if foot positioning is correct
    if foot_prev >= foot
        flag_foot_position = 1;
    else
        flag_foot_position = 0;
    end
    
end

end

== matlab function vslipsl_sim/Triggered Subsystem/SLIP-SL controller ==
  data: X input; U output; flag input; ref_star_ss input; ref_star_ds input; gains input; param input; ref_output_ss output; ref_output_ds output; det_A_ss output; K_ss output; error_ss output; Lie_f_h output; Lie2_f_h output; det_A_ds output
function [U, ref_output_ss, ref_output_ds, det_A_ss, K_ss, error_ss, Lie_f_h, Lie2_f_h, det_A_ds] = fcn(X, flag, ref_star_ss, ref_star_ds, gains, param)

% ----------- parameters ----------------------
L0_ss = param(1); % [m]
k0_ss = param(2); % nominal leg stiffness [N/m]
m_M = param(3); % hip mass [kg]
m_swLeg = param(4); % [kg]
m_swFoot = param(5); % [kg]
I_swLeg = param(6); %
I_swFoot = param(7); %
L_thigh = param(8); % [m]
k_swFoot = param(9); %
k_swLeg = param(10); %
theta0 = param(11); %[rad]
r0 = param(12); % [m]
gravi = param(13); % gravitational acc

L0_ds = param(14); % [m] free length of the springs in the DS
k0_ds = param(15); % [N/m] stiffness of the springs in the DS

% ----------- flags ----------------------
f_stance = flag(1); % indicates which stance phase it is
foot = flag(2); % location of the stance foot
foot_prev = flag(3) - foot; % previous location of the stance foot
x_CoM_TD = flag(4) - foot; % x_CoM @TD
x_CoM_LO = flag(5); % x_CoM @LO
flag_ref_ob = flag(6); % raised if ref. state var. starts out of bounds at stage trans.

% ----------- states ----------------------
x_M = X(1) - foot; % x position of main mass in SS
y_M = X(2); % z position of main mass in SS
theta = X(3); % angle of the swing leg when in SS
r = X(4); % distance of the foot from the knee on SS
x_CoM = X(5) - foot; % x position of the CoM
y_CoM = X(6);

dx_M = X(7); % x velocity of main mass in SS
dy_M = X(8); % z velocity of main mass in SS
dtheta = X(9);
dr = X(10);
dx_CoM = X(11);
dy_CoM = X(12);

q = [x_M; y_M; theta; r; x_CoM; y_CoM];
dq = [dx_M; dy_M; dtheta; dr; dx_CoM; dy_CoM];

%---------- controller -----------------------------

% SS inputs
u1 = 0; % input for stance leg spring
u2 = 0; % input for swing leg torsional spring
u3 = 0; % input for swing foot spring
% DS inputs
u4 = 0; % input for stance leg spring
u5 = 0; % input for swing leg spring

% Controller Gains
K_p = gains(1);
K_d = gains(2);

K_p_sw = gains(3);
K_d_sw = gains(4);

K_p_ds = gains(5);
K_d_ds = gains(6);
K_v_ds = gains(7); % 5 in visser 2012

% for debugging
ref_output_ss = [0; 0; 0];
det_A_ss = NaN;
K_ss = [NaN; NaN; NaN];
error_ss = [NaN; NaN; NaN];
Lie_f_h = [NaN; NaN; NaN];
Lie2_f_h = [NaN; NaN; NaN];

ref_output_ds = [0;0];
det_A_ds = 0;

x_CoM_star_ss = ref_star_ss(:,11);
x_CoM_star_ds = ref_star_ds(:,1);

%%

if f_stance == 1
    % if the system is in single stance phase

    % Calculating the phase variable x_CoM
    x_swLeg = x_M + (L_thigh/2)*cos(theta);
    x_swFoot = x_M + (L_thigh + r)*cos(theta);
    x_CoM = (m_M*x_M + m_swLeg*x_swLeg + m_swFoot*x_swFoot)/(m_M + m_swLeg + m_swFoot);

    if x_CoM_star_ss(1) <= x_CoM && x_CoM <= x_CoM_star_ss(end)

        % testing function implementation
        X_slipsl_ss = [x_M; y_M; theta; r; dx_M; dy_M; dtheta; dr];
        [U_ss, det_A_ss, K_ss, error_ss, Lie_f_h, Lie2_f_h] = VSLIPSL_SS_controller( ...
            x_CoM, X_slipsl_ss, ref_star_ss, param, gains);

        u1 = U_ss(1);
        u2 = U_ss(2);
        u3 = U_ss(3);

    else
        ref_output_ss = [-1; -1; -1];
    end

else
    % if the system is in double stance phace

    if x_CoM_star_ds(1) <= x_CoM && x_CoM <= x_CoM_star_ds(end)
    % if x_CoM <= x_CoM_star_ds(end)

        % interpolation
        y_CoM_star = interp1(x_CoM_star_ds, ref_star_ds(:,2), x_CoM);
        dx_CoM_star = interp1(x_CoM_star_ds, ref_star_ds(:,3), x_CoM);

        del_y_CoM_star = interp1(x_CoM_star_ds, ref_star_ds(:,4), x_CoM);
        del_dx_CoM_star = interp1(x_CoM_star_ds, ref_star_ds(:,5), x_CoM);

        del2_y_CoM_star = interp1(x_CoM_star_ds, ref_star_ds(:,6), x_CoM);

        ref_output_ds = [y_CoM_star; dx_CoM_star];

        A_ds = [
            ((y_CoM - del_y_CoM_star*x_CoM)*(L0_ds - (x_CoM^2 + y_CoM^2)^(1/2)))/((x_CoM^2 + y_CoM^2)^(1/2)*(m_M + m_swLeg + m_swFoot)), (y_CoM*(L0_ds/(y_CoM^2 + (foot_prev - x_CoM)^2)^(1/2) - 1))/(m_M + m_swLeg + m_swFoot) + (del_y_CoM_star*(foot_prev - x_CoM)*(L0_ds/(y_CoM^2 + (foot_prev - x_CoM)^2)^(1/2) - 1))/(m_M + m_swLeg + m_swFoot)
            (x_CoM*(L0_ds/(x_CoM^2 + y_CoM^2)^(1/2) - 1))/(m_M + m_swLeg + m_swFoot),                                                                                                        -((foot_prev - x_CoM)*(L0_ds/(y_CoM^2 + (foot_prev - x_CoM)^2)^(1/2) - 1))/(m_M + m_swLeg + m_swFoot)];

        K_ds = [
            del2_y_CoM_star*dx_CoM^2 - K_p_ds*(y_CoM - y_CoM_star) - K_d_ds*(dy_CoM - del_y_CoM_star*dx_CoM) - (k0_ds*y_CoM*(L0_ds/(x_CoM^2 + y_CoM^2)^(1/2) - 1) - gravi*(m_M + m_swLeg + m_swFoot) + k0_ds*y_CoM*(L0_ds/(y_CoM^2 + (foot_prev - x_CoM)^2)^(1/2) - 1))/(m_M + m_swLeg + m_swFoot) - (del_y_CoM_star*(k0_ds*(foot_prev - x_CoM)*(L0_ds/(y_CoM^2 + (foot_prev - x_CoM)^2)^(1/2) - 1) - k0_ds*x_CoM*(L0_ds/(x_CoM^2 + y_CoM^2)^(1/2) - 1)))/(m_M + m_swLeg + m_swFoot);
            del_dx_CoM_star*dx_CoM - K_v_ds*(dx_CoM - dx_CoM_star) + (k0_ds*(foot_prev - x_CoM)*(L0_ds/(y_CoM^2 + (foot_prev - x_CoM)^2)^(1/2) - 1) - k0_ds*x_CoM*(L0_ds/(x_CoM^2 + y_CoM^2)^(1/2) - 1))/(m_M + m_swLeg + m_swFoot)];

        % % regularization terms
        % eps_ds = 5e-5;
        % eps_4 = eps_ds/det(A_ds);
        % eps_5 = eps_ds/det(A_ds);
        %
        % E_ds = [1/(eps_4 + 1), 0; 0, 1/(eps_5 + 1)];
        %
        % U_ds = E_ds*(A_ds^-1)*K_ds;

        det_A_ds = det(A_ds);

        % if abs(det_A_ds) >= 1e-9
        if abs(det_A_ds) >= 4e-9
            U_ds = (A_ds^-1)*K_ds;
            u4 = U_ds(1);
            u5 = U_ds(2);
        else
            u4 = 0;
            u5 = 0;
        end

    end

end

U = [u1; u2; u3; u4; u5];

% clipped = max(min(x, upper), lower);
var_stiff_bound_cst = 0.5;
upper = (1 + var_stiff_bound_cst);
lower = (var_stiff_bound_cst - 1);
U = [
    max(min(u1, k0_ss*upper), k0_ss*lower);
    max(min(u2, k_swLeg*upper), k_swLeg*lower);
    max(min(u3, k_swFoot*upper), k_swFoot*lower);
    max(min(u4, k0_ds*upper), k0_ds*lower);
    max(min(u5, k0_ds*upper), k0_ds*lower)];
